simulink library "Miscellaneous"  (Simulink 8.7)
settings: Solver=ode45  StartTime=0.0  StopTime=10.0  RelTol=1e-3
undefined symbols (not defined in the file): c
libraries: Memory_Blocks_Lib x100, Bit_Multiplexers_Lib x35, simulink_extras x13, commutil2 x10, Decoders_Lib x7
settings Model: Creator=N  LastModifiedBy=Jozko Mrkvicka

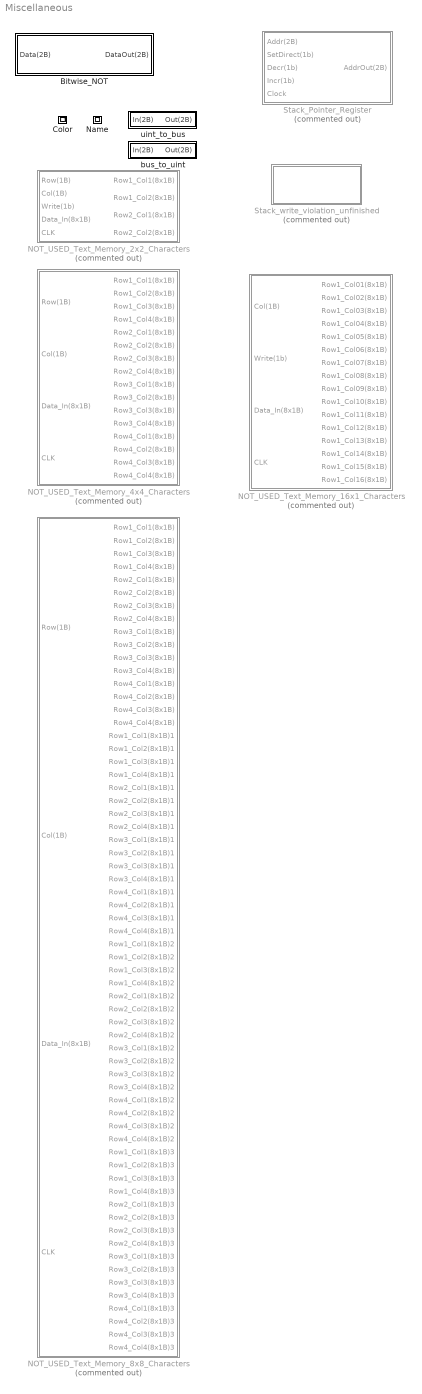
== system Miscellaneous ==
  Bitwise_NOT : Subsystem
  Color : Subsystem
  NOT_USED_Text_Memory_16x1_Characters : Subsystem  Commented=on
  NOT_USED_Text_Memory_2x2_Characters : Subsystem  Commented=on
  NOT_USED_Text_Memory_4x4_Characters : Subsystem  Commented=on
  NOT_USED_Text_Memory_8x8_Characters : Subsystem  Commented=on
  Name : Subsystem
  Stack_Pointer_Register : Subsystem  Commented=on
  Stack_write_violation_unfinished : Subsystem  Commented=on
  bus_to_uint : Subsystem
  uint_to_bus : Subsystem

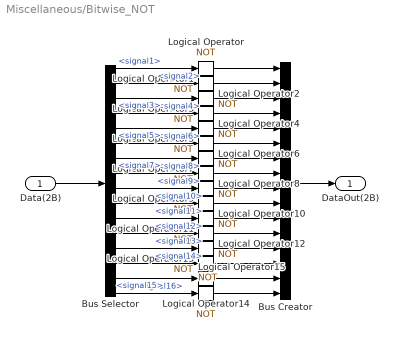
== system Miscellaneous/Bitwise_NOT ==
  Data(2B) : Inport
  Bus Creator : BusCreator  Inputs=16
  Bus Selector : BusSelector  OutputSignals=signal1,signal2,signal3,signal4,signal5,signal6,signal7,signal8,signal9,signal10,signal11,signal12,signal13,signal14,signal15,signal16
  Logical Operator{,1..15} (16 alike) : Logic  Operator=NOT  IconShape=distinctive  AllPortsSameDT=off  OutDataTypeStr=boolean
  DataOut(2B) : Outport
  wires:
  Bus Creator/1 -> DataOut(2B)/1
  Data(2B)/1 -> Bus Selector/1
  Logical Operator/1 -> Bus Creator/1
  Logical Operator1/1 -> Bus Creator/2
  Logical Operator2/1 -> Bus Creator/3
  Logical Operator7/1 -> Bus Creator/8
  Logical Operator6/1 -> Bus Creator/7
  Logical Operator5/1 -> Bus Creator/6
  Logical Operator3/1 -> Bus Creator/4
  Logical Operator4/1 -> Bus Creator/5
  Bus Selector/8 -> Logical Operator7/1  "<signal8>"
  Bus Selector/7 -> Logical Operator6/1  "<signal7>"
  Bus Selector/6 -> Logical Operator5/1  "<signal6>"
  Bus Selector/5 -> Logical Operator4/1  "<signal5>"
  Bus Selector/4 -> Logical Operator3/1  "<signal4>"
  Bus Selector/3 -> Logical Operator2/1  "<signal3>"
  Bus Selector/2 -> Logical Operator1/1  "<signal2>"
  Bus Selector/1 -> Logical Operator/1  "<signal1>"
  Bus Selector/16 -> Logical Operator15/1  "<signal16>"
  Bus Selector/15 -> Logical Operator14/1  "<signal15>"
  Bus Selector/14 -> Logical Operator13/1  "<signal14>"
  Bus Selector/13 -> Logical Operator12/1  "<signal13>"
  Bus Selector/12 -> Logical Operator11/1  "<signal12>"
  Bus Selector/11 -> Logical Operator10/1  "<signal11>"
  Bus Selector/10 -> Logical Operator9/1  "<signal10>"
  Bus Selector/9 -> Logical Operator8/1  "<signal9>"
  Logical Operator8/1 -> Bus Creator/9
  Logical Operator9/1 -> Bus Creator/10
  Logical Operator10/1 -> Bus Creator/11
  Logical Operator11/1 -> Bus Creator/12
  Logical Operator12/1 -> Bus Creator/13
  Logical Operator13/1 -> Bus Creator/14
  Logical Operator14/1 -> Bus Creator/15
  Logical Operator15/1 -> Bus Creator/16

== system Miscellaneous/Color ==
  note: This block is just a workaround for changing color of a line which is connected to it (Simulink does not allow to assign colors to particular lines).
  " " : Inport
  "  " : Outport
  wires:
  " "/1 -> "  "/1

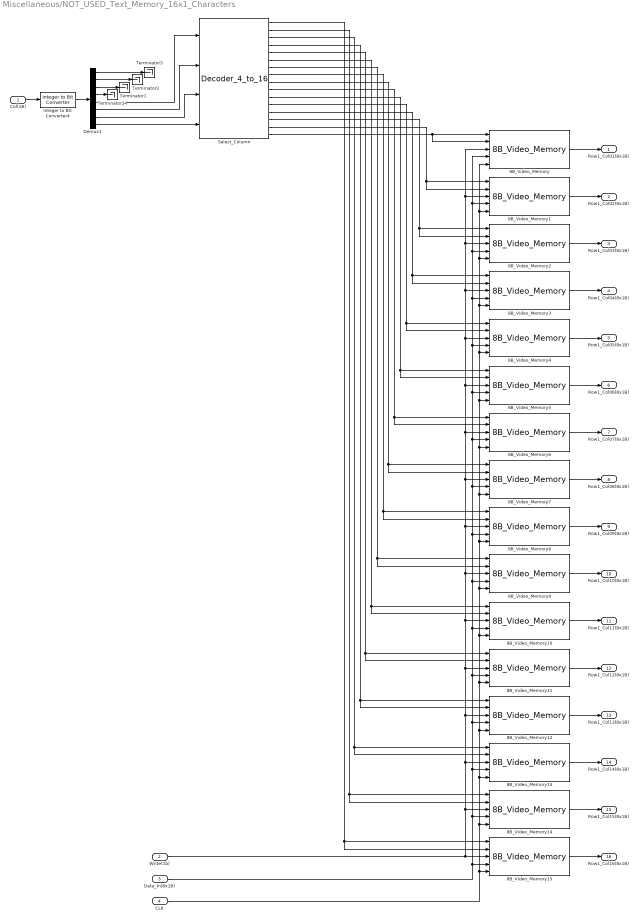
== system Miscellaneous/NOT_USED_Text_Memory_16x1_Characters ==
  Col(1B) : Inport
  Write(1b) : Inport  Port=2
  Data_In(8x1B) : Inport  Port=3
  CLK : Inport  Port=4
  8B_Video_Memory{,1..15} (16 alike) : Memory_Blocks_Lib/Memory_Blocks_Lib/8B_Video_Memory
  Demux1 : Demux  Outputs=8
  Integer to Bit Converter4 : commutil2/Integer to Bit Converter  nbits=8  signedInputValues=Unsigned  bitOrder=MSB first  outDtype=uint8
  Select_Column : Decoders_Lib/Decoders_Lib/Decoder_4_to_16
  Terminator{1..3,24} (4 alike) : Terminator
  Row1_Col01(8x1B) : Outport
  Row1_Col02(8x1B) : Outport  Port=2
  Row1_Col03(8x1B) : Outport  Port=3
  Row1_Col04(8x1B) : Outport  Port=4
  Row1_Col05(8x1B) : Outport  Port=5
  Row1_Col06(8x1B) : Outport  Port=6
  Row1_Col07(8x1B) : Outport  Port=7
  Row1_Col08(8x1B) : Outport  Port=8
  Row1_Col09(8x1B) : Outport  Port=9
  Row1_Col10(8x1B) : Outport  Port=10
  Row1_Col11(8x1B) : Outport  Port=11
  Row1_Col12(8x1B) : Outport  Port=12
  Row1_Col13(8x1B) : Outport  Port=13
  Row1_Col14(8x1B) : Outport  Port=14
  Row1_Col15(8x1B) : Outport  Port=15
  Row1_Col16(8x1B) : Outport  Port=16
  wires:
  Col(1B)/1 -> Integer to Bit Converter4/1
  Integer to Bit Converter4/1 -> Demux1/1
  Data_In(8x1B)/1 -> 8B_Video_Memory6/4, 8B_Video_Memory5/4, 8B_Video_Memory4/4, 8B_Video_Memory3/4, 8B_Video_Memory2/4, 8B_Video_Memory/4, 8B_Video_Memory1/4, 8B_Video_Memory7/4, 8B_Video_Memory8/4, 8B_Video_Memory9/4, 8B_Video_Memory10/4, 8B_Video_Memory11/4, 8B_Video_Memory12/4, 8B_Video_Memory13/4, 8B_Video_Memory14/4, 8B_Video_Memory15/4
  8B_Video_Memory/1 -> Row1_Col01(8x1B)/1
  8B_Video_Memory1/1 -> Row1_Col02(8x1B)/1
  8B_Video_Memory2/1 -> Row1_Col03(8x1B)/1
  8B_Video_Memory3/1 -> Row1_Col04(8x1B)/1
  CLK/1 -> 8B_Video_Memory6/5, 8B_Video_Memory5/5, 8B_Video_Memory4/5, 8B_Video_Memory3/5, 8B_Video_Memory2/5, 8B_Video_Memory/5, 8B_Video_Memory1/5, 8B_Video_Memory7/5, 8B_Video_Memory8/5, 8B_Video_Memory9/5, 8B_Video_Memory10/5, 8B_Video_Memory11/5, 8B_Video_Memory12/5, 8B_Video_Memory13/5, 8B_Video_Memory14/5, 8B_Video_Memory15/5
  8B_Video_Memory4/1 -> Row1_Col05(8x1B)/1
  8B_Video_Memory5/1 -> Row1_Col06(8x1B)/1
  8B_Video_Memory6/1 -> Row1_Col07(8x1B)/1
  8B_Video_Memory7/1 -> Row1_Col08(8x1B)/1
  8B_Video_Memory8/1 -> Row1_Col09(8x1B)/1
  8B_Video_Memory9/1 -> Row1_Col10(8x1B)/1
  8B_Video_Memory10/1 -> Row1_Col11(8x1B)/1
  8B_Video_Memory11/1 -> Row1_Col12(8x1B)/1
  8B_Video_Memory12/1 -> Row1_Col13(8x1B)/1
  8B_Video_Memory13/1 -> Row1_Col14(8x1B)/1
  8B_Video_Memory14/1 -> Row1_Col15(8x1B)/1
  8B_Video_Memory15/1 -> Row1_Col16(8x1B)/1
  Demux1/5 -> Select_Column/1
  Demux1/6 -> Select_Column/2
  Demux1/8 -> Select_Column/4
  Demux1/7 -> Select_Column/3
  Select_Column/16 -> 8B_Video_Memory/2, 8B_Video_Memory/1
  Select_Column/15 -> 8B_Video_Memory1/2, 8B_Video_Memory1/1
  Write(1b)/1 -> 8B_Video_Memory/3, 8B_Video_Memory1/3, 8B_Video_Memory2/3, 8B_Video_Memory3/3, 8B_Video_Memory4/3, 8B_Video_Memory5/3, 8B_Video_Memory6/3, 8B_Video_Memory7/3, 8B_Video_Memory8/3, 8B_Video_Memory9/3, 8B_Video_Memory10/3, 8B_Video_Memory11/3, 8B_Video_Memory12/3, 8B_Video_Memory13/3, 8B_Video_Memory14/3, 8B_Video_Memory15/3
  Select_Column/14 -> 8B_Video_Memory2/2, 8B_Video_Memory2/1
  Select_Column/13 -> 8B_Video_Memory3/1, 8B_Video_Memory3/2
  Select_Column/12 -> 8B_Video_Memory4/1, 8B_Video_Memory4/2
  Select_Column/11 -> 8B_Video_Memory5/1, 8B_Video_Memory5/2
  Select_Column/10 -> 8B_Video_Memory6/1, 8B_Video_Memory6/2
  Select_Column/9 -> 8B_Video_Memory7/1, 8B_Video_Memory7/2
  Select_Column/8 -> 8B_Video_Memory8/1, 8B_Video_Memory8/2
  Select_Column/7 -> 8B_Video_Memory9/1, 8B_Video_Memory9/2
  Select_Column/6 -> 8B_Video_Memory10/1, 8B_Video_Memory10/2
  Select_Column/5 -> 8B_Video_Memory11/1, 8B_Video_Memory11/2
  Select_Column/4 -> 8B_Video_Memory12/1, 8B_Video_Memory12/2
  Select_Column/3 -> 8B_Video_Memory13/1, 8B_Video_Memory13/2
  Select_Column/2 -> 8B_Video_Memory14/1, 8B_Video_Memory14/2
  Select_Column/1 -> 8B_Video_Memory15/1, 8B_Video_Memory15/2
  Demux1/4 -> Terminator24/1
  Demux1/3 -> Terminator1/1
  Demux1/2 -> Terminator2/1
  Demux1/1 -> Terminator3/1

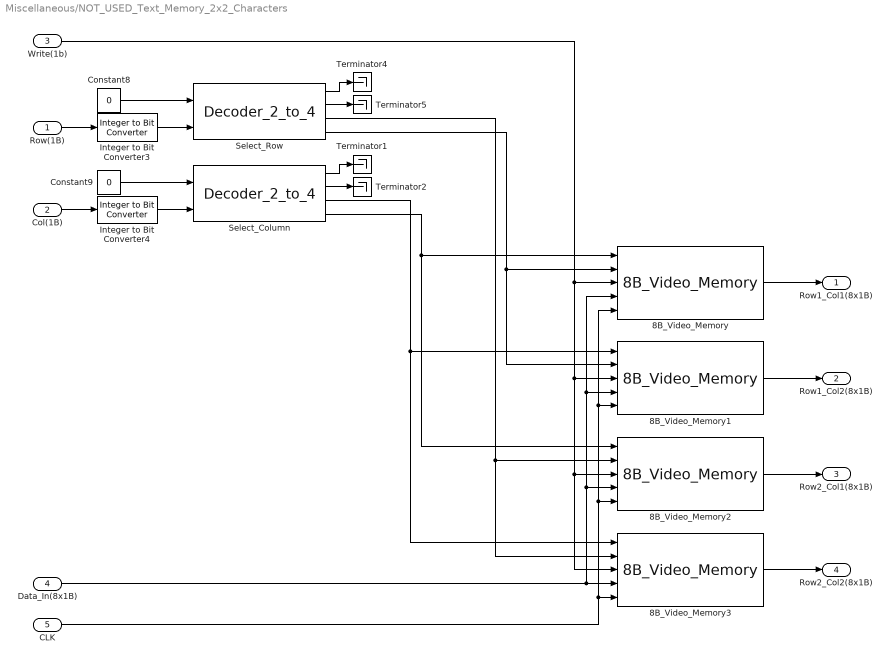
== system Miscellaneous/NOT_USED_Text_Memory_2x2_Characters ==
  Row(1B) : Inport
  Col(1B) : Inport  Port=2
  Write(1b) : Inport  Port=3
  Data_In(8x1B) : Inport  Port=4
  CLK : Inport  Port=5
  8B_Video_Memory{,1..3} (4 alike) : Memory_Blocks_Lib/Memory_Blocks_Lib/8B_Video_Memory
  Constant8 : Constant  Value=0  OutDataTypeStr=uint8
  Constant9 : Constant  Value=0  OutDataTypeStr=uint8
  Integer to Bit Converter3 : commutil2/Integer to Bit Converter  nbits=1  signedInputValues=Unsigned  bitOrder=MSB first  outDtype=uint8
  Integer to Bit Converter4 : commutil2/Integer to Bit Converter  nbits=1  signedInputValues=Unsigned  bitOrder=MSB first  outDtype=uint8
  Select_Column : Decoders_Lib/Decoders_Lib/Decoder_2_to_4
  Select_Row : Decoders_Lib/Decoders_Lib/Decoder_2_to_4
  Terminator{1..2,4..5} (4 alike) : Terminator
  Row1_Col1(8x1B) : Outport
  Row1_Col2(8x1B) : Outport  Port=2
  Row2_Col1(8x1B) : Outport  Port=3
  Row2_Col2(8x1B) : Outport  Port=4
  wires:
  Row(1B)/1 -> Integer to Bit Converter3/1
  Integer to Bit Converter3/1 -> Select_Row/2
  Constant8/1 -> Select_Row/1
  Constant9/1 -> Select_Column/1
  Col(1B)/1 -> Integer to Bit Converter4/1
  Integer to Bit Converter4/1 -> Select_Column/2
  Data_In(8x1B)/1 -> 8B_Video_Memory/4, 8B_Video_Memory1/4, 8B_Video_Memory2/4, 8B_Video_Memory3/4
  8B_Video_Memory/1 -> Row1_Col1(8x1B)/1
  8B_Video_Memory1/1 -> Row1_Col2(8x1B)/1
  8B_Video_Memory2/1 -> Row2_Col1(8x1B)/1
  8B_Video_Memory3/1 -> Row2_Col2(8x1B)/1
  CLK/1 -> 8B_Video_Memory/5, 8B_Video_Memory1/5, 8B_Video_Memory2/5, 8B_Video_Memory3/5
  Select_Row/1 -> Terminator4/1
  Select_Row/2 -> Terminator5/1
  Select_Column/1 -> Terminator1/1
  Select_Column/2 -> Terminator2/1
  Select_Row/4 -> 8B_Video_Memory1/2, 8B_Video_Memory/2
  Select_Row/3 -> 8B_Video_Memory3/2, 8B_Video_Memory2/2
  Select_Column/4 -> 8B_Video_Memory2/1, 8B_Video_Memory/1
  Select_Column/3 -> 8B_Video_Memory3/1, 8B_Video_Memory1/1
  Write(1b)/1 -> 8B_Video_Memory/3, 8B_Video_Memory1/3, 8B_Video_Memory2/3, 8B_Video_Memory3/3

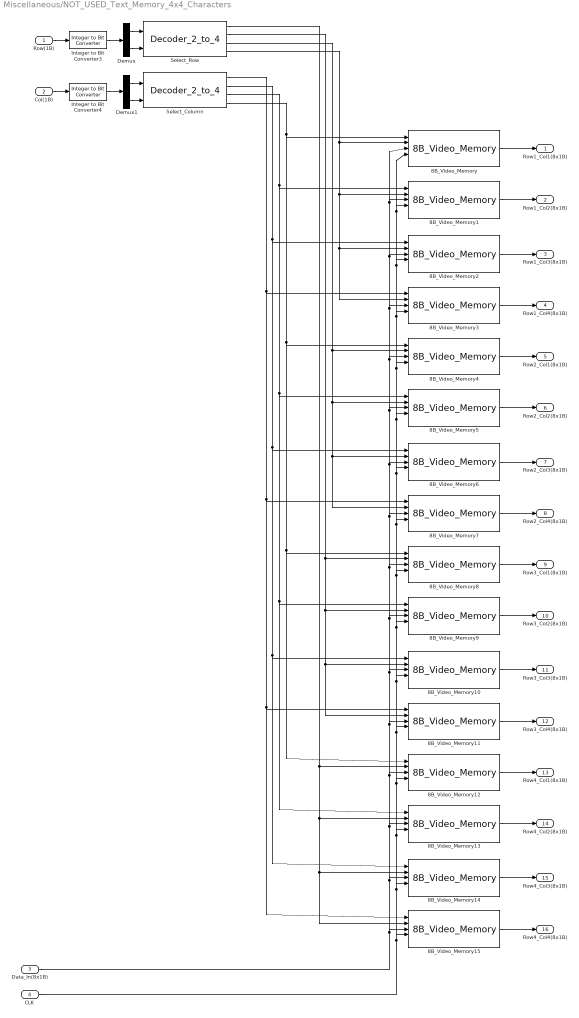
== system Miscellaneous/NOT_USED_Text_Memory_4x4_Characters ==
  Row(1B) : Inport
  Col(1B) : Inport  Port=2
  Data_In(8x1B) : Inport  Port=3
  CLK : Inport  Port=4
  8B_Video_Memory{,1..15} (16 alike) : Memory_Blocks_Lib/Memory_Blocks_Lib/8B_Video_Memory
  Demux : Demux  Outputs=2
  Demux1 : Demux  Outputs=2
  Integer to Bit Converter3 : commutil2/Integer to Bit Converter  nbits=2  signedInputValues=Unsigned  bitOrder=MSB first  outDtype=uint8
  Integer to Bit Converter4 : commutil2/Integer to Bit Converter  nbits=2  signedInputValues=Unsigned  bitOrder=MSB first  outDtype=uint8
  Select_Column : Decoders_Lib/Decoders_Lib/Decoder_2_to_4
  Select_Row : Decoders_Lib/Decoders_Lib/Decoder_2_to_4
  Row1_Col1(8x1B) : Outport
  Row1_Col2(8x1B) : Outport  Port=2
  Row1_Col3(8x1B) : Outport  Port=3
  Row1_Col4(8x1B) : Outport  Port=4
  Row2_Col1(8x1B) : Outport  Port=5
  Row2_Col2(8x1B) : Outport  Port=6
  Row2_Col3(8x1B) : Outport  Port=7
  Row2_Col4(8x1B) : Outport  Port=8
  Row3_Col1(8x1B) : Outport  Port=9
  Row3_Col2(8x1B) : Outport  Port=10
  Row3_Col3(8x1B) : Outport  Port=11
  Row3_Col4(8x1B) : Outport  Port=12
  Row4_Col1(8x1B) : Outport  Port=13
  Row4_Col2(8x1B) : Outport  Port=14
  Row4_Col3(8x1B) : Outport  Port=15
  Row4_Col4(8x1B) : Outport  Port=16
  wires:
  Row(1B)/1 -> Integer to Bit Converter3/1
  Integer to Bit Converter3/1 -> Demux/1
  Col(1B)/1 -> Integer to Bit Converter4/1
  Integer to Bit Converter4/1 -> Demux1/1
  Data_In(8x1B)/1 -> 8B_Video_Memory15/3, 8B_Video_Memory14/3, 8B_Video_Memory13/3, 8B_Video_Memory12/3, 8B_Video_Memory11/3, 8B_Video_Memory10/3, 8B_Video_Memory9/3, 8B_Video_Memory8/3, 8B_Video_Memory6/3, 8B_Video_Memory5/3, 8B_Video_Memory4/3, 8B_Video_Memory2/3, 8B_Video_Memory1/3, 8B_Video_Memory/3, 8B_Video_Memory3/3, 8B_Video_Memory7/3
  8B_Video_Memory/1 -> Row1_Col1(8x1B)/1
  8B_Video_Memory1/1 -> Row1_Col2(8x1B)/1
  8B_Video_Memory2/1 -> Row1_Col3(8x1B)/1
  8B_Video_Memory3/1 -> Row1_Col4(8x1B)/1
  CLK/1 -> 8B_Video_Memory15/4, 8B_Video_Memory14/4, 8B_Video_Memory13/4, 8B_Video_Memory12/4, 8B_Video_Memory11/4, 8B_Video_Memory10/4, 8B_Video_Memory9/4, 8B_Video_Memory8/4, 8B_Video_Memory7/4, 8B_Video_Memory6/4, 8B_Video_Memory5/4, 8B_Video_Memory4/4, 8B_Video_Memory3/4, 8B_Video_Memory2/4, 8B_Video_Memory1/4, 8B_Video_Memory/4
  Select_Row/1 -> 8B_Video_Memory12/2, 8B_Video_Memory13/2, 8B_Video_Memory14/2, 8B_Video_Memory15/2
  Select_Row/2 -> 8B_Video_Memory8/2, 8B_Video_Memory9/2, 8B_Video_Memory10/2, 8B_Video_Memory11/2
  Select_Column/1 -> 8B_Video_Memory15/1, 8B_Video_Memory11/1, 8B_Video_Memory7/1, 8B_Video_Memory3/1
  Select_Column/2 -> 8B_Video_Memory14/1, 8B_Video_Memory10/1, 8B_Video_Memory6/1, 8B_Video_Memory2/1
  Select_Row/4 -> 8B_Video_Memory/2, 8B_Video_Memory1/2, 8B_Video_Memory2/2, 8B_Video_Memory3/2
  Select_Row/3 -> 8B_Video_Memory4/2, 8B_Video_Memory5/2, 8B_Video_Memory6/2, 8B_Video_Memory7/2
  Select_Column/4 -> 8B_Video_Memory12/1, 8B_Video_Memory8/1, 8B_Video_Memory4/1, 8B_Video_Memory/1
  Select_Column/3 -> 8B_Video_Memory13/1, 8B_Video_Memory9/1, 8B_Video_Memory5/1, 8B_Video_Memory1/1
  8B_Video_Memory4/1 -> Row2_Col1(8x1B)/1
  8B_Video_Memory5/1 -> Row2_Col2(8x1B)/1
  8B_Video_Memory6/1 -> Row2_Col3(8x1B)/1
  8B_Video_Memory7/1 -> Row2_Col4(8x1B)/1
  8B_Video_Memory8/1 -> Row3_Col1(8x1B)/1
  8B_Video_Memory9/1 -> Row3_Col2(8x1B)/1
  8B_Video_Memory10/1 -> Row3_Col3(8x1B)/1
  8B_Video_Memory11/1 -> Row3_Col4(8x1B)/1
  8B_Video_Memory12/1 -> Row4_Col1(8x1B)/1
  8B_Video_Memory13/1 -> Row4_Col2(8x1B)/1
  8B_Video_Memory14/1 -> Row4_Col3(8x1B)/1
  8B_Video_Memory15/1 -> Row4_Col4(8x1B)/1
  Demux/1 -> Select_Row/1
  Demux/2 -> Select_Row/2
  Demux1/1 -> Select_Column/1
  Demux1/2 -> Select_Column/2

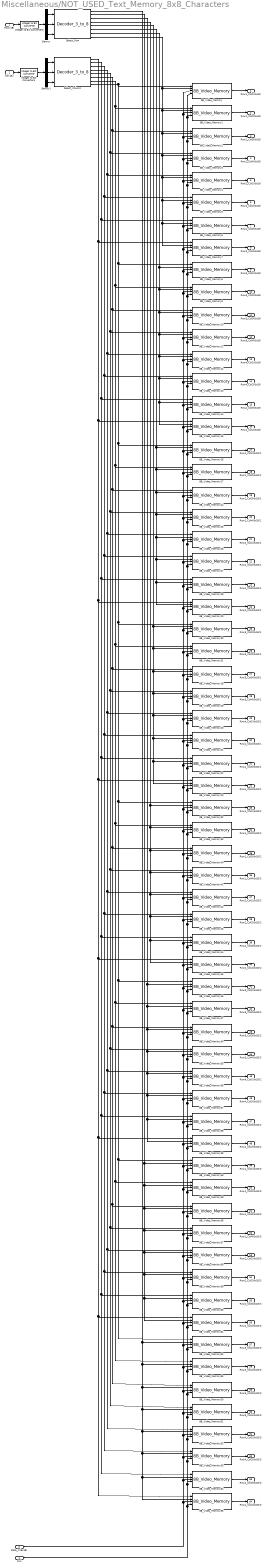
== system Miscellaneous/NOT_USED_Text_Memory_8x8_Characters ==
  Row(1B) : Inport
  Col(1B) : Inport  Port=2
  Data_In(8x1B) : Inport  Port=3
  CLK : Inport  Port=4
  8B_Video_Memory{,1..63} (64 alike) : Memory_Blocks_Lib/Memory_Blocks_Lib/8B_Video_Memory
  Demux : Demux  Outputs=3
  Demux1 : Demux  Outputs=3
  Integer to Bit Converter3 : commutil2/Integer to Bit Converter  nbits=3  signedInputValues=Unsigned  bitOrder=MSB first  outDtype=uint8
  Integer to Bit Converter4 : commutil2/Integer to Bit Converter  nbits=3  signedInputValues=Unsigned  bitOrder=MSB first  outDtype=uint8
  Select_Column : Decoders_Lib/Decoders_Lib/Decoder_3_to_8
  Select_Row : Decoders_Lib/Decoders_Lib/Decoder_3_to_8
  Row1_Col1(8x1B) : Outport
  Row1_Col2(8x1B) : Outport  Port=2
  Row1_Col3(8x1B) : Outport  Port=3
  Row1_Col4(8x1B) : Outport  Port=4
  Row2_Col1(8x1B) : Outport  Port=5
  Row2_Col2(8x1B) : Outport  Port=6
  Row2_Col3(8x1B) : Outport  Port=7
  Row2_Col4(8x1B) : Outport  Port=8
  Row3_Col1(8x1B) : Outport  Port=9
  Row3_Col2(8x1B) : Outport  Port=10
  Row3_Col3(8x1B) : Outport  Port=11
  Row3_Col4(8x1B) : Outport  Port=12
  Row4_Col1(8x1B) : Outport  Port=13
  Row4_Col2(8x1B) : Outport  Port=14
  Row4_Col3(8x1B) : Outport  Port=15
  Row4_Col4(8x1B) : Outport  Port=16
  Row1_Col1(8x1B)1 : Outport  Port=17
  Row1_Col2(8x1B)1 : Outport  Port=18
  Row1_Col3(8x1B)1 : Outport  Port=19
  Row1_Col4(8x1B)1 : Outport  Port=20
  Row2_Col1(8x1B)1 : Outport  Port=21
  Row2_Col2(8x1B)1 : Outport  Port=22
  Row2_Col3(8x1B)1 : Outport  Port=23
  Row2_Col4(8x1B)1 : Outport  Port=24
  Row3_Col1(8x1B)1 : Outport  Port=25
  Row3_Col2(8x1B)1 : Outport  Port=26
  Row3_Col3(8x1B)1 : Outport  Port=27
  Row3_Col4(8x1B)1 : Outport  Port=28
  Row4_Col1(8x1B)1 : Outport  Port=29
  Row4_Col2(8x1B)1 : Outport  Port=30
  Row4_Col3(8x1B)1 : Outport  Port=31
  Row4_Col4(8x1B)1 : Outport  Port=32
  Row1_Col1(8x1B)2 : Outport  Port=33
  Row1_Col2(8x1B)2 : Outport  Port=34
  Row1_Col3(8x1B)2 : Outport  Port=35
  Row1_Col4(8x1B)2 : Outport  Port=36
  Row2_Col1(8x1B)2 : Outport  Port=37
  Row2_Col2(8x1B)2 : Outport  Port=38
  Row2_Col3(8x1B)2 : Outport  Port=39
  Row2_Col4(8x1B)2 : Outport  Port=40
  Row3_Col1(8x1B)2 : Outport  Port=41
  Row3_Col2(8x1B)2 : Outport  Port=42
  Row3_Col3(8x1B)2 : Outport  Port=43
  Row3_Col4(8x1B)2 : Outport  Port=44
  Row4_Col1(8x1B)2 : Outport  Port=45
  Row4_Col2(8x1B)2 : Outport  Port=46
  Row4_Col3(8x1B)2 : Outport  Port=47
  Row4_Col4(8x1B)2 : Outport  Port=48
  Row1_Col1(8x1B)3 : Outport  Port=49
  Row1_Col2(8x1B)3 : Outport  Port=50
  Row1_Col3(8x1B)3 : Outport  Port=51
  Row1_Col4(8x1B)3 : Outport  Port=52
  Row2_Col1(8x1B)3 : Outport  Port=53
  Row2_Col2(8x1B)3 : Outport  Port=54
  Row2_Col3(8x1B)3 : Outport  Port=55
  Row2_Col4(8x1B)3 : Outport  Port=56
  Row3_Col1(8x1B)3 : Outport  Port=57
  Row3_Col2(8x1B)3 : Outport  Port=58
  Row3_Col3(8x1B)3 : Outport  Port=59
  Row3_Col4(8x1B)3 : Outport  Port=60
  Row4_Col1(8x1B)3 : Outport  Port=61
  Row4_Col2(8x1B)3 : Outport  Port=62
  Row4_Col3(8x1B)3 : Outport  Port=63
  Row4_Col4(8x1B)3 : Outport  Port=64
  wires:
  Row(1B)/1 -> Integer to Bit Converter3/1
  Integer to Bit Converter3/1 -> Demux/1
  Col(1B)/1 -> Integer to Bit Converter4/1
  Integer to Bit Converter4/1 -> Demux1/1
  8B_Video_Memory/1 -> Row1_Col1(8x1B)/1
  8B_Video_Memory1/1 -> Row1_Col2(8x1B)/1
  8B_Video_Memory2/1 -> Row1_Col3(8x1B)/1
  8B_Video_Memory3/1 -> Row1_Col4(8x1B)/1
  Select_Row/5 -> 8B_Video_Memory30/2, 8B_Video_Memory31/2, 8B_Video_Memory18/2, 8B_Video_Memory19/2, 8B_Video_Memory20/2, 8B_Video_Memory21/2, 8B_Video_Memory22/2, 8B_Video_Memory23/2
  Select_Row/6 -> 8B_Video_Memory16/2, 8B_Video_Memory17/2, 8B_Video_Memory24/2, 8B_Video_Memory25/2, 8B_Video_Memory26/2, 8B_Video_Memory27/2, 8B_Video_Memory28/2, 8B_Video_Memory29/2
  Select_Column/5 -> 8B_Video_Memory3/1, 8B_Video_Memory51/1, 8B_Video_Memory57/1, 8B_Video_Memory35/1, 8B_Video_Memory41/1, 8B_Video_Memory19/1, 8B_Video_Memory25/1, 8B_Video_Memory11/1
  Select_Column/6 -> 8B_Video_Memory2/1, 8B_Video_Memory50/1, 8B_Video_Memory56/1, 8B_Video_Memory34/1, 8B_Video_Memory40/1, 8B_Video_Memory18/1, 8B_Video_Memory24/1, 8B_Video_Memory10/1
  Select_Row/8 -> 8B_Video_Memory/2, 8B_Video_Memory1/2, 8B_Video_Memory2/2, 8B_Video_Memory3/2, 8B_Video_Memory4/2, 8B_Video_Memory5/2, 8B_Video_Memory6/2, 8B_Video_Memory7/2
  Select_Row/7 -> 8B_Video_Memory8/2, 8B_Video_Memory9/2, 8B_Video_Memory10/2, 8B_Video_Memory11/2, 8B_Video_Memory12/2, 8B_Video_Memory13/2, 8B_Video_Memory14/2, 8B_Video_Memory15/2
  Select_Column/8 -> 8B_Video_Memory/1, 8B_Video_Memory62/1, 8B_Video_Memory48/1, 8B_Video_Memory46/1, 8B_Video_Memory32/1, 8B_Video_Memory30/1, 8B_Video_Memory16/1, 8B_Video_Memory8/1
  Select_Column/7 -> 8B_Video_Memory1/1, 8B_Video_Memory63/1, 8B_Video_Memory49/1, 8B_Video_Memory47/1, 8B_Video_Memory33/1, 8B_Video_Memory31/1, 8B_Video_Memory17/1, 8B_Video_Memory9/1
  8B_Video_Memory4/1 -> Row2_Col1(8x1B)/1
  8B_Video_Memory5/1 -> Row2_Col2(8x1B)/1
  8B_Video_Memory6/1 -> Row2_Col3(8x1B)/1
  8B_Video_Memory7/1 -> Row2_Col4(8x1B)/1
  8B_Video_Memory8/1 -> Row3_Col1(8x1B)/1
  8B_Video_Memory9/1 -> Row3_Col2(8x1B)/1
  8B_Video_Memory10/1 -> Row3_Col3(8x1B)/1
  8B_Video_Memory11/1 -> Row3_Col4(8x1B)/1
  8B_Video_Memory12/1 -> Row4_Col1(8x1B)/1
  8B_Video_Memory13/1 -> Row4_Col2(8x1B)/1
  8B_Video_Memory14/1 -> Row4_Col3(8x1B)/1
  8B_Video_Memory15/1 -> Row4_Col4(8x1B)/1
  Demux/1 -> Select_Row/1
  Demux/2 -> Select_Row/2
  Demux1/1 -> Select_Column/1
  Demux1/2 -> Select_Column/2
  8B_Video_Memory16/1 -> Row1_Col1(8x1B)1/1
  8B_Video_Memory17/1 -> Row1_Col2(8x1B)1/1
  8B_Video_Memory24/1 -> Row1_Col3(8x1B)1/1
  8B_Video_Memory25/1 -> Row1_Col4(8x1B)1/1
  8B_Video_Memory26/1 -> Row2_Col1(8x1B)1/1
  8B_Video_Memory27/1 -> Row2_Col2(8x1B)1/1
  8B_Video_Memory28/1 -> Row2_Col3(8x1B)1/1
  8B_Video_Memory29/1 -> Row2_Col4(8x1B)1/1
  8B_Video_Memory30/1 -> Row3_Col1(8x1B)1/1
  8B_Video_Memory31/1 -> Row3_Col2(8x1B)1/1
  8B_Video_Memory18/1 -> Row3_Col3(8x1B)1/1
  8B_Video_Memory19/1 -> Row3_Col4(8x1B)1/1
  8B_Video_Memory20/1 -> Row4_Col1(8x1B)1/1
  8B_Video_Memory21/1 -> Row4_Col2(8x1B)1/1
  8B_Video_Memory22/1 -> Row4_Col3(8x1B)1/1
  8B_Video_Memory23/1 -> Row4_Col4(8x1B)1/1
  8B_Video_Memory32/1 -> Row1_Col1(8x1B)2/1
  8B_Video_Memory33/1 -> Row1_Col2(8x1B)2/1
  8B_Video_Memory40/1 -> Row1_Col3(8x1B)2/1
  8B_Video_Memory41/1 -> Row1_Col4(8x1B)2/1
  8B_Video_Memory42/1 -> Row2_Col1(8x1B)2/1
  8B_Video_Memory43/1 -> Row2_Col2(8x1B)2/1
  8B_Video_Memory44/1 -> Row2_Col3(8x1B)2/1
  8B_Video_Memory45/1 -> Row2_Col4(8x1B)2/1
  8B_Video_Memory46/1 -> Row3_Col1(8x1B)2/1
  8B_Video_Memory47/1 -> Row3_Col2(8x1B)2/1
  8B_Video_Memory34/1 -> Row3_Col3(8x1B)2/1
  8B_Video_Memory35/1 -> Row3_Col4(8x1B)2/1
  8B_Video_Memory36/1 -> Row4_Col1(8x1B)2/1
  8B_Video_Memory37/1 -> Row4_Col2(8x1B)2/1
  8B_Video_Memory38/1 -> Row4_Col3(8x1B)2/1
  8B_Video_Memory39/1 -> Row4_Col4(8x1B)2/1
  8B_Video_Memory48/1 -> Row1_Col1(8x1B)3/1
  8B_Video_Memory49/1 -> Row1_Col2(8x1B)3/1
  8B_Video_Memory56/1 -> Row1_Col3(8x1B)3/1
  8B_Video_Memory57/1 -> Row1_Col4(8x1B)3/1
  8B_Video_Memory58/1 -> Row2_Col1(8x1B)3/1
  8B_Video_Memory59/1 -> Row2_Col2(8x1B)3/1
  8B_Video_Memory60/1 -> Row2_Col3(8x1B)3/1
  8B_Video_Memory61/1 -> Row2_Col4(8x1B)3/1
  8B_Video_Memory62/1 -> Row3_Col1(8x1B)3/1
  8B_Video_Memory63/1 -> Row3_Col2(8x1B)3/1
  8B_Video_Memory50/1 -> Row3_Col3(8x1B)3/1
  8B_Video_Memory51/1 -> Row3_Col4(8x1B)3/1
  8B_Video_Memory52/1 -> Row4_Col1(8x1B)3/1
  8B_Video_Memory53/1 -> Row4_Col2(8x1B)3/1
  8B_Video_Memory54/1 -> Row4_Col3(8x1B)3/1
  8B_Video_Memory55/1 -> Row4_Col4(8x1B)3/1
  Data_In(8x1B)/1 -> 8B_Video_Memory55/3, 8B_Video_Memory54/3, 8B_Video_Memory53/3, 8B_Video_Memory52/3, 8B_Video_Memory51/3, 8B_Video_Memory50/3, 8B_Video_Memory63/3, 8B_Video_Memory62/3, 8B_Video_Memory61/3, 8B_Video_Memory60/3, 8B_Video_Memory59/3, 8B_Video_Memory58/3, 8B_Video_Memory57/3, 8B_Video_Memory56/3, 8B_Video_Memory49/3, 8B_Video_Memory48/3, 8B_Video_Memory39/3, 8B_Video_Memory38/3, 8B_Video_Memory37/3, 8B_Video_Memory36/3, 8B_Video_Memory35/3, 8B_Video_Memory34/3, 8B_Video_Memory47/3, 8B_Video_Memory46/3, 8B_Video_Memory45/3, 8B_Video_Memory44/3, 8B_Video_Memory43/3, 8B_Video_Memory42/3, 8B_Video_Memory41/3, 8B_Video_Memory40/3, 8B_Video_Memory33/3, 8B_Video_Memory32/3, 8B_Video_Memory23/3, 8B_Video_Memory22/3, 8B_Video_Memory21/3, 8B_Video_Memory20/3, 8B_Video_Memory19/3, 8B_Video_Memory18/3, 8B_Video_Memory31/3, 8B_Video_Memory30/3, 8B_Video_Memory29/3, 8B_Video_Memory28/3, 8B_Video_Memory27/3, 8B_Video_Memory26/3, 8B_Video_Memory25/3, 8B_Video_Memory24/3, 8B_Video_Memory17/3, 8B_Video_Memory16/3, 8B_Video_Memory15/3, 8B_Video_Memory14/3, 8B_Video_Memory13/3, 8B_Video_Memory12/3, 8B_Video_Memory11/3, 8B_Video_Memory10/3, 8B_Video_Memory9/3, 8B_Video_Memory8/3, 8B_Video_Memory6/3, 8B_Video_Memory5/3, 8B_Video_Memory4/3, 8B_Video_Memory2/3, 8B_Video_Memory1/3, 8B_Video_Memory/3, 8B_Video_Memory3/3, 8B_Video_Memory7/3
  CLK/1 -> 8B_Video_Memory55/4, 8B_Video_Memory54/4, 8B_Video_Memory53/4, 8B_Video_Memory52/4, 8B_Video_Memory51/4, 8B_Video_Memory50/4, 8B_Video_Memory63/4, 8B_Video_Memory62/4, 8B_Video_Memory61/4, 8B_Video_Memory60/4, 8B_Video_Memory59/4, 8B_Video_Memory58/4, 8B_Video_Memory57/4, 8B_Video_Memory56/4, 8B_Video_Memory49/4, 8B_Video_Memory48/4, 8B_Video_Memory39/4, 8B_Video_Memory38/4, 8B_Video_Memory37/4, 8B_Video_Memory36/4, 8B_Video_Memory35/4, 8B_Video_Memory34/4, 8B_Video_Memory47/4, 8B_Video_Memory46/4, 8B_Video_Memory45/4, 8B_Video_Memory44/4, 8B_Video_Memory43/4, 8B_Video_Memory42/4, 8B_Video_Memory41/4, 8B_Video_Memory40/4, 8B_Video_Memory33/4, 8B_Video_Memory32/4, 8B_Video_Memory23/4, 8B_Video_Memory22/4, 8B_Video_Memory21/4, 8B_Video_Memory20/4, 8B_Video_Memory19/4, 8B_Video_Memory18/4, 8B_Video_Memory31/4, 8B_Video_Memory30/4, 8B_Video_Memory29/4, 8B_Video_Memory28/4, 8B_Video_Memory27/4, 8B_Video_Memory26/4, 8B_Video_Memory25/4, 8B_Video_Memory24/4, 8B_Video_Memory17/4, 8B_Video_Memory16/4, 8B_Video_Memory15/4, 8B_Video_Memory14/4, 8B_Video_Memory13/4, 8B_Video_Memory12/4, 8B_Video_Memory11/4, 8B_Video_Memory10/4, 8B_Video_Memory9/4, 8B_Video_Memory8/4, 8B_Video_Memory7/4, 8B_Video_Memory6/4, 8B_Video_Memory5/4, 8B_Video_Memory4/4, 8B_Video_Memory3/4, 8B_Video_Memory2/4, 8B_Video_Memory1/4, 8B_Video_Memory/4
  Select_Row/4 -> 8B_Video_Memory32/2, 8B_Video_Memory33/2, 8B_Video_Memory40/2, 8B_Video_Memory41/2, 8B_Video_Memory42/2, 8B_Video_Memory43/2, 8B_Video_Memory44/2, 8B_Video_Memory45/2
  Select_Row/3 -> 8B_Video_Memory46/2, 8B_Video_Memory47/2, 8B_Video_Memory34/2, 8B_Video_Memory35/2, 8B_Video_Memory36/2, 8B_Video_Memory37/2, 8B_Video_Memory38/2, 8B_Video_Memory39/2
  Select_Row/2 -> 8B_Video_Memory48/2, 8B_Video_Memory49/2, 8B_Video_Memory56/2, 8B_Video_Memory57/2, 8B_Video_Memory58/2, 8B_Video_Memory60/2, 8B_Video_Memory61/2, 8B_Video_Memory59/2
  Select_Row/1 -> 8B_Video_Memory62/2, 8B_Video_Memory63/2, 8B_Video_Memory50/2, 8B_Video_Memory51/2, 8B_Video_Memory52/2, 8B_Video_Memory53/2, 8B_Video_Memory54/2, 8B_Video_Memory55/2
  Select_Column/4 -> 8B_Video_Memory52/1, 8B_Video_Memory58/1, 8B_Video_Memory36/1, 8B_Video_Memory42/1, 8B_Video_Memory20/1, 8B_Video_Memory26/1, 8B_Video_Memory12/1, 8B_Video_Memory4/1
  Select_Column/3 -> 8B_Video_Memory53/1, 8B_Video_Memory59/1, 8B_Video_Memory37/1, 8B_Video_Memory43/1, 8B_Video_Memory21/1, 8B_Video_Memory27/1, 8B_Video_Memory13/1, 8B_Video_Memory5/1
  Select_Column/2 -> 8B_Video_Memory54/1, 8B_Video_Memory60/1, 8B_Video_Memory38/1, 8B_Video_Memory44/1, 8B_Video_Memory22/1, 8B_Video_Memory28/1, 8B_Video_Memory14/1, 8B_Video_Memory6/1
  Select_Column/1 -> 8B_Video_Memory55/1, 8B_Video_Memory61/1, 8B_Video_Memory39/1, 8B_Video_Memory45/1, 8B_Video_Memory23/1, 8B_Video_Memory29/1, 8B_Video_Memory15/1, 8B_Video_Memory7/1
  Demux/3 -> Select_Row/3
  Demux1/3 -> Select_Column/3

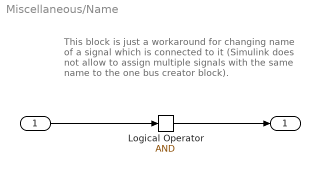
== system Miscellaneous/Name ==
  note: This block is just a workaround for changing name of a signal which is connected to it (Simulink does not allow to assign multiple signals with the same name to the one bus creator block).
  " " : Inport
  Logical Operator : Logic  Inputs=1  IconShape=distinctive  AllPortsSameDT=off  OutDataTypeStr=boolean
  "  " : Outport
  wires:
  " "/1 -> Logical Operator/1
  Logical Operator/1 -> "  "/1

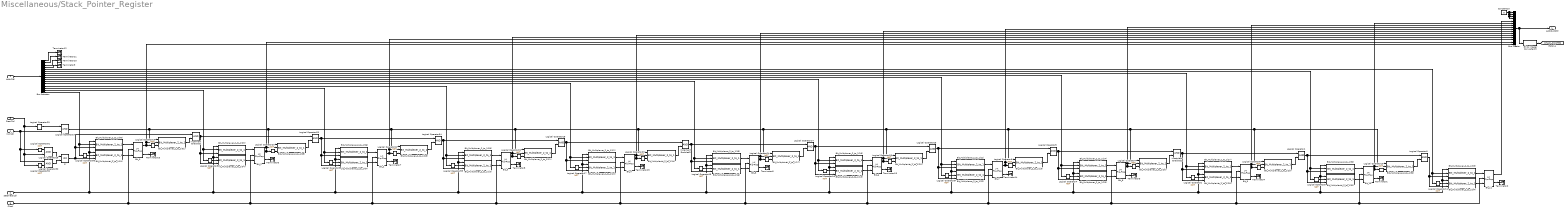
== system Miscellaneous/Stack_Pointer_Register ==
  Addr(2B) : Inport
  SetDirect(1b) : Inport  Port=2
  Decr(1b) : Inport  Port=3
  Incr(1b) : Inport  Port=4
  Clock : Inport  Port=5
  Bit to Integer Converter15 : commutil2/Bit to Integer Converter  nbits=16  bitOrder=MSB first  signedOutputValues=Unsigned  outDtype=uint16  outDtypeSigned=Inherit via internal rule
  Bit_0 : simulink_extras/Flip Flops/J-K Flip-Flop  initial_condition=bitand(c.STACK_START, bin2dec('0000 0000 0001'))
  Bit_1 : simulink_extras/Flip Flops/J-K Flip-Flop  initial_condition=bitand(c.STACK_START, bin2dec('0000 0000 0010'))
  Bit_10 : simulink_extras/Flip Flops/J-K Flip-Flop  initial_condition=bitand(c.STACK_START, bin2dec('0100 0000 0000'))
  Bit_11 : simulink_extras/Flip Flops/J-K Flip-Flop  initial_condition=bitand(c.STACK_START, bin2dec('1000 0000 0000'))
  Bit_2 : simulink_extras/Flip Flops/J-K Flip-Flop  initial_condition=bitand(c.STACK_START, bin2dec('0000 0000 0100'))
  Bit_3 : simulink_extras/Flip Flops/J-K Flip-Flop  initial_condition=bitand(c.STACK_START, bin2dec('0000 0000 1000'))
  Bit_4 : simulink_extras/Flip Flops/J-K Flip-Flop  initial_condition=bitand(c.STACK_START, bin2dec('0000 0001 0000'))
  Bit_5 : simulink_extras/Flip Flops/J-K Flip-Flop  initial_condition=bitand(c.STACK_START, bin2dec('0000 0010 0000'))
  Bit_6 : simulink_extras/Flip Flops/J-K Flip-Flop  initial_condition=bitand(c.STACK_START, bin2dec('0000 0100 0000'))
  Bit_7 : simulink_extras/Flip Flops/J-K Flip-Flop  initial_condition=bitand(c.STACK_START, bin2dec('0000 1000 0000'))
  Bit_8 : simulink_extras/Flip Flops/J-K Flip-Flop  initial_condition=bitand(c.STACK_START, bin2dec('0001 0000 0000'))
  Bit_9 : simulink_extras/Flip Flops/J-K Flip-Flop  initial_condition=bitand(c.STACK_START, bin2dec('0010 0000 0000'))
  Bit_Multiplexer_2_to_1(00) : Bit_Multiplexers_Lib/Bit_Multiplexers_Lib/Bit_Multiplexer_2_to_1
  Bit_Multiplexer_2_to_1(01) : Bit_Multiplexers_Lib/Bit_Multiplexers_Lib/Bit_Multiplexer_2_to_1
  Bit_Multiplexer_2_to_1(02) : Bit_Multiplexers_Lib/Bit_Multiplexers_Lib/Bit_Multiplexer_2_to_1
  Bit_Multiplexer_2_to_1(03) : Bit_Multiplexers_Lib/Bit_Multiplexers_Lib/Bit_Multiplexer_2_to_1
  Bit_Multiplexer_2_to_1(04) : Bit_Multiplexers_Lib/Bit_Multiplexers_Lib/Bit_Multiplexer_2_to_1
  Bit_Multiplexer_2_to_1(05) : Bit_Multiplexers_Lib/Bit_Multiplexers_Lib/Bit_Multiplexer_2_to_1
  Bit_Multiplexer_2_to_1(06) : Bit_Multiplexers_Lib/Bit_Multiplexers_Lib/Bit_Multiplexer_2_to_1
  Bit_Multiplexer_2_to_1(07) : Bit_Multiplexers_Lib/Bit_Multiplexers_Lib/Bit_Multiplexer_2_to_1
  Bit_Multiplexer_2_to_1(08) : Bit_Multiplexers_Lib/Bit_Multiplexers_Lib/Bit_Multiplexer_2_to_1
  Bit_Multiplexer_2_to_1(09) : Bit_Multiplexers_Lib/Bit_Multiplexers_Lib/Bit_Multiplexer_2_to_1
  Bit_Multiplexer_2_to_1(10) : Bit_Multiplexers_Lib/Bit_Multiplexers_Lib/Bit_Multiplexer_2_to_1
  Bit_Multiplexer_2_to_1(11) : Bit_Multiplexers_Lib/Bit_Multiplexers_Lib/Bit_Multiplexer_2_to_1
  Bit_Multiplexer_2_to_1(12) : Bit_Multiplexers_Lib/Bit_Multiplexers_Lib/Bit_Multiplexer_2_to_1
  Bit_Multiplexer_2_to_1(13) : Bit_Multiplexers_Lib/Bit_Multiplexers_Lib/Bit_Multiplexer_2_to_1
  Bit_Multiplexer_2_to_1(14) : Bit_Multiplexers_Lib/Bit_Multiplexers_Lib/Bit_Multiplexer_2_to_1
  Bit_Multiplexer_2_to_1(15) : Bit_Multiplexers_Lib/Bit_Multiplexers_Lib/Bit_Multiplexer_2_to_1
  Bit_Multiplexer_2_to_1(16) : Bit_Multiplexers_Lib/Bit_Multiplexers_Lib/Bit_Multiplexer_2_to_1
  Bit_Multiplexer_2_to_1(17) : Bit_Multiplexers_Lib/Bit_Multiplexers_Lib/Bit_Multiplexer_2_to_1
  Bit_Multiplexer_2_to_1(18) : Bit_Multiplexers_Lib/Bit_Multiplexers_Lib/Bit_Multiplexer_2_to_1
  Bit_Multiplexer_2_to_1(19) : Bit_Multiplexers_Lib/Bit_Multiplexers_Lib/Bit_Multiplexer_2_to_1
  Bit_Multiplexer_2_to_1(20) : Bit_Multiplexers_Lib/Bit_Multiplexers_Lib/Bit_Multiplexer_2_to_1
  Bit_Multiplexer_2_to_1(21) : Bit_Multiplexers_Lib/Bit_Multiplexers_Lib/Bit_Multiplexer_2_to_1
  Bit_Multiplexer_2_to_1(22) : Bit_Multiplexers_Lib/Bit_Multiplexers_Lib/Bit_Multiplexer_2_to_1
  Bit_Multiplexer_2_to_1(23) : Bit_Multiplexers_Lib/Bit_Multiplexers_Lib/Bit_Multiplexer_2_to_1
  Bit_Multiplexer_2_to_1(24) : Bit_Multiplexers_Lib/Bit_Multiplexers_Lib/Bit_Multiplexer_2_to_1
  Bit_Multiplexer_2_to_1(25) : Bit_Multiplexers_Lib/Bit_Multiplexers_Lib/Bit_Multiplexer_2_to_1
  Bit_Multiplexer_2_to_1(26) : Bit_Multiplexers_Lib/Bit_Multiplexers_Lib/Bit_Multiplexer_2_to_1
  Bit_Multiplexer_2_to_1(27) : Bit_Multiplexers_Lib/Bit_Multiplexers_Lib/Bit_Multiplexer_2_to_1
  Bit_Multiplexer_2_to_1(28) : Bit_Multiplexers_Lib/Bit_Multiplexers_Lib/Bit_Multiplexer_2_to_1
  Bit_Multiplexer_2_to_1(29) : Bit_Multiplexers_Lib/Bit_Multiplexers_Lib/Bit_Multiplexer_2_to_1
  Bit_Multiplexer_2_to_1(30) : Bit_Multiplexers_Lib/Bit_Multiplexers_Lib/Bit_Multiplexer_2_to_1
  Bit_Multiplexer_2_to_1(31) : Bit_Multiplexers_Lib/Bit_Multiplexers_Lib/Bit_Multiplexer_2_to_1
  Bit_Multiplexer_2_to_1(32) : Bit_Multiplexers_Lib/Bit_Multiplexers_Lib/Bit_Multiplexer_2_to_1
  Bit_Multiplexer_2_to_1(33) : Bit_Multiplexers_Lib/Bit_Multiplexers_Lib/Bit_Multiplexer_2_to_1
  Bit_Multiplexer_2_to_1(34) : Bit_Multiplexers_Lib/Bit_Multiplexers_Lib/Bit_Multiplexer_2_to_1
  Bus Creator : BusCreator  Inputs=16
  Bus Selector : BusSelector  OutputSignals=signal1,signal2,signal3,signal4,signal5,signal6,signal7,signal8,signal9,signal10,signal11,signal12,signal13,signal14,signal15,signal16
  Constant10 : Constant  Value=0  OutDataTypeStr=boolean
  Increment Enabled1 : Logic  IconShape=distinctive  AllPortsSameDT=off  OutDataTypeStr=boolean
  Increment Enabled2 : Logic  IconShape=distinctive  AllPortsSameDT=off  OutDataTypeStr=boolean
  Increment Enabled3 : Logic  IconShape=distinctive  AllPortsSameDT=off  OutDataTypeStr=boolean
  Logical Operator{1,5,9,14,18,25,27..28,30,33..34} (11 alike) : Logic  IconShape=distinctive  AllPortsSameDT=off  OutDataTypeStr=boolean
  Logical Operator{2..4,6..8,10..11,15..17,19..24,26,29,31..32,35..39} (26 alike) : Logic  Operator=NOT  IconShape=distinctive  AllPortsSameDT=off  OutDataTypeStr=boolean
  Terminator{1..16} (16 alike) : Terminator
  or : Logic  Operator=OR  IconShape=distinctive  AllPortsSameDT=off  OutDataTypeStr=boolean
  AddrOut(2B) : Outport
  tag scope: STACK_POINTER=global
  wires:
  Logical Operator18/1 -> Increment Enabled3/1, Bit_Multiplexer_2_to_1(13)/3, Bit_Multiplexer_2_to_1(12)/3
  Bus Selector/12 -> Bit_Multiplexer_2_to_1(12)/2, Logical Operator17/1  "<signal12>"
  Logical Operator17/1 -> Bit_Multiplexer_2_to_1(13)/2
  Bit_4/1 -> Bus Creator/12, Bit_Multiplexer_2_to_1(14)/2, Logical Operator23/1
  Bus Selector/9 -> Bit_Multiplexer_2_to_1(21)/2, Logical Operator37/1  "<signal9>"
  Logical Operator37/1 -> Bit_Multiplexer_2_to_1(22)/2
  Bit_Multiplexer_2_to_1(21)/1 -> Bit_7/1
  Bit_Multiplexer_2_to_1(22)/1 -> Bit_7/3
  Logical Operator16/1 -> Bit_Multiplexer_2_to_1(19)/2
  Bus Selector/10 -> Bit_Multiplexer_2_to_1(18)/2, Logical Operator16/1  "<signal10>"
  Bit_Multiplexer_2_to_1(19)/1 -> Bit_6/3
  Bit_Multiplexer_2_to_1(18)/1 -> Bit_6/1
  Bus Selector/11 -> Bit_Multiplexer_2_to_1(15)/2, Logical Operator15/1  "<signal11>"
  Logical Operator15/1 -> Bit_Multiplexer_2_to_1(16)/2
  Bit_Multiplexer_2_to_1(16)/1 -> Bit_5/3
  Bit_Multiplexer_2_to_1(15)/1 -> Bit_5/1
  Bit_Multiplexer_2_to_1(12)/1 -> Bit_4/1
  Bit_Multiplexer_2_to_1(13)/1 -> Bit_4/3
  Bit_7/1 -> Bus Creator/9, Bit_Multiplexer_2_to_1(23)/2, Logical Operator6/1
  Bit_6/1 -> Bus Creator/10, Bit_Multiplexer_2_to_1(20)/2, Logical Operator26/1
  Bit_7/2 -> Terminator14/1
  Logical Operator14/1 -> Logical Operator25/1, Bit_Multiplexer_2_to_1(19)/3, Bit_Multiplexer_2_to_1(18)/3
  Bit_5/1 -> Bus Creator/11, Bit_Multiplexer_2_to_1(17)/2, Logical Operator24/1
  Increment Enabled3/1 -> Logical Operator14/1, Bit_Multiplexer_2_to_1(16)/3, Bit_Multiplexer_2_to_1(15)/3
  Bit_6/2 -> Terminator13/1
  Bit_5/2 -> Terminator5/1
  Bit_4/2 -> Terminator15/1
  Logical Operator34/1 -> Logical Operator18/1, Bit_Multiplexer_2_to_1(10)/3, Bit_Multiplexer_2_to_1(09)/3
  Bit_0/1 -> Bus Creator/16, Bit_Multiplexer_2_to_1(02)/2, Logical Operator19/1
  Bus Selector/13 -> Logical Operator35/1, Bit_Multiplexer_2_to_1(09)/2  "<signal13>"
  Logical Operator35/1 -> Bit_Multiplexer_2_to_1(10)/2
  Bit_Multiplexer_2_to_1(09)/1 -> Bit_3/1
  Bit_Multiplexer_2_to_1(10)/1 -> Bit_3/3
  Logical Operator39/1 -> Bit_Multiplexer_2_to_1(07)/2
  Bus Selector/14 -> Logical Operator39/1, Bit_Multiplexer_2_to_1(06)/2  "<signal14>"
  Bit_Multiplexer_2_to_1(07)/1 -> Bit_2/3
  Bit_Multiplexer_2_to_1(06)/1 -> Bit_2/1
  Bus Selector/15 -> Logical Operator38/1, Bit_Multiplexer_2_to_1(03)/2  "<signal15>"
  Logical Operator38/1 -> Bit_Multiplexer_2_to_1(04)/2
  Bit_Multiplexer_2_to_1(04)/1 -> Bit_1/3
  Bit_Multiplexer_2_to_1(03)/1 -> Bit_1/1
  Logical Operator36/1 -> Bit_Multiplexer_2_to_1(01)/2
  Bit_Multiplexer_2_to_1(00)/1 -> Bit_0/1
  Bit_Multiplexer_2_to_1(01)/1 -> Bit_0/3
  Bus Selector/16 -> Logical Operator36/1, Bit_Multiplexer_2_to_1(00)/2  "<signal16>"
  Addr(2B)/1 -> Bus Selector/1
  Bit_3/1 -> Bus Creator/13, Bit_Multiplexer_2_to_1(11)/2, Logical Operator22/1
  Bit_2/1 -> Bus Creator/14, Bit_Multiplexer_2_to_1(08)/2, Logical Operator21/1
  Bit_3/2 -> Terminator8/1
  Logical Operator33/1 -> Logical Operator34/1, Bit_Multiplexer_2_to_1(07)/3, Bit_Multiplexer_2_to_1(06)/3
  Bit_1/1 -> Bus Creator/15, Bit_Multiplexer_2_to_1(05)/2, Logical Operator20/1
  Increment Enabled2/1 -> Bit_Multiplexer_2_to_1(04)/3, Bit_Multiplexer_2_to_1(03)/3, Logical Operator33/1
  Bit_2/2 -> Terminator7/1
  Bit_1/2 -> Terminator6/1
  Bit_0/2 -> Terminator16/1
  or/1 -> Bit_Multiplexer_2_to_1(01)/3, Increment Enabled2/1, Bit_Multiplexer_2_to_1(00)/3
  Logical Operator19/1 -> Bit_Multiplexer_2_to_1(02)/3
  Logical Operator20/1 -> Bit_Multiplexer_2_to_1(05)/3
  Logical Operator21/1 -> Bit_Multiplexer_2_to_1(08)/3
  Logical Operator22/1 -> Bit_Multiplexer_2_to_1(11)/3
  Logical Operator23/1 -> Bit_Multiplexer_2_to_1(14)/3
  Logical Operator24/1 -> Bit_Multiplexer_2_to_1(17)/3
  Logical Operator26/1 -> Bit_Multiplexer_2_to_1(20)/3
  Logical Operator29/1 -> Logical Operator27/1
  Bit_Multiplexer_2_to_1(02)/1 -> Increment Enabled2/2
  Bit_Multiplexer_2_to_1(05)/1 -> Logical Operator33/2
  Bit_Multiplexer_2_to_1(08)/1 -> Logical Operator34/2
  Bit_Multiplexer_2_to_1(11)/1 -> Logical Operator18/2
  Bit_Multiplexer_2_to_1(14)/1 -> Increment Enabled3/2
  Bit_Multiplexer_2_to_1(17)/1 -> Logical Operator14/2
  Bit_Multiplexer_2_to_1(20)/1 -> Logical Operator25/2
  Logical Operator28/1 -> or/1
  Logical Operator30/1 -> or/2
  Logical Operator31/1 -> Logical Operator28/1
  Decr(1b)/1 -> Logical Operator32/1, Logical Operator28/2, Logical Operator29/1
  Incr(1b)/1 -> Logical Operator27/2, Logical Operator30/1, Logical Operator31/1
  Logical Operator32/1 -> Logical Operator30/2
  Bus Creator/1 -> Bit to Integer Converter15/1, AddrOut(2B)/1
  Logical Operator5/1 -> Increment Enabled1/1, Bit_Multiplexer_2_to_1(25)/3, Bit_Multiplexer_2_to_1(24)/3
  Bus Selector/8 -> Bit_Multiplexer_2_to_1(24)/2, Logical Operator4/1  "<signal8>"
  Logical Operator4/1 -> Bit_Multiplexer_2_to_1(25)/2
  Bit_8/1 -> Bus Creator/8, Bit_Multiplexer_2_to_1(26)/2, Logical Operator7/1
  Bus Selector/5 -> Bit_Multiplexer_2_to_1(33)/2, Logical Operator11/1  "<signal5>"
  Logical Operator11/1 -> Bit_Multiplexer_2_to_1(34)/2
  Bit_Multiplexer_2_to_1(33)/1 -> Bit_11/1
  Bit_Multiplexer_2_to_1(34)/1 -> Bit_11/3
  Logical Operator3/1 -> Bit_Multiplexer_2_to_1(31)/2
  Bus Selector/6 -> Bit_Multiplexer_2_to_1(30)/2, Logical Operator3/1  "<signal6>"
  Bit_Multiplexer_2_to_1(31)/1 -> Bit_10/3
  Bit_Multiplexer_2_to_1(30)/1 -> Bit_10/1
  Bus Selector/7 -> Bit_Multiplexer_2_to_1(27)/2, Logical Operator2/1  "<signal7>"
  Logical Operator2/1 -> Bit_Multiplexer_2_to_1(28)/2
  Bit_Multiplexer_2_to_1(28)/1 -> Bit_9/3
  Bit_Multiplexer_2_to_1(27)/1 -> Bit_9/1
  SetDirect(1b)/1 -> Bit_Multiplexer_2_to_1(01)/1, Bit_Multiplexer_2_to_1(00)/1, Bit_Multiplexer_2_to_1(04)/1, Bit_Multiplexer_2_to_1(03)/1, Bit_Multiplexer_2_to_1(07)/1, Bit_Multiplexer_2_to_1(06)/1, Bit_Multiplexer_2_to_1(10)/1, Bit_Multiplexer_2_to_1(09)/1, Bit_Multiplexer_2_to_1(13)/1, Bit_Multiplexer_2_to_1(12)/1, Bit_Multiplexer_2_to_1(16)/1, Bit_Multiplexer_2_to_1(15)/1, Bit_Multiplexer_2_to_1(19)/1, Bit_Multiplexer_2_to_1(18)/1, Bit_Multiplexer_2_to_1(22)/1, Bit_Multiplexer_2_to_1(21)/1, Bit_Multiplexer_2_to_1(25)/1, Bit_Multiplexer_2_to_1(24)/1, Bit_Multiplexer_2_to_1(28)/1, Bit_Multiplexer_2_to_1(27)/1, Bit_Multiplexer_2_to_1(31)/1, Bit_Multiplexer_2_to_1(30)/1, Bit_Multiplexer_2_to_1(34)/1, Bit_Multiplexer_2_to_1(33)/1
  Bit_Multiplexer_2_to_1(24)/1 -> Bit_8/1
  Bit_Multiplexer_2_to_1(25)/1 -> Bit_8/3
  Bit_11/1 -> Bus Creator/5
  Bit_10/1 -> Bus Creator/6, Bit_Multiplexer_2_to_1(32)/2, Logical Operator10/1
  Logical Operator9/1 -> Bit_Multiplexer_2_to_1(34)/3, Bit_Multiplexer_2_to_1(33)/3
  Bit_11/2 -> Terminator2/1
  Logical Operator1/1 -> Logical Operator9/1, Bit_Multiplexer_2_to_1(31)/3, Bit_Multiplexer_2_to_1(30)/3
  Bit_9/1 -> Bus Creator/7, Bit_Multiplexer_2_to_1(29)/2, Logical Operator8/1
  Increment Enabled1/1 -> Logical Operator1/1, Bit_Multiplexer_2_to_1(28)/3, Bit_Multiplexer_2_to_1(27)/3
  Bit_10/2 -> Terminator1/1
  Clock/1 -> Bit_0/2, Bit_1/2, Bit_2/2, Bit_3/2, Bit_4/2, Bit_5/2, Bit_6/2, Bit_7/2, Bit_8/2, Bit_9/2, Bit_10/2, Bit_11/2
  Bit_9/2 -> Terminator4/1
  Bit_8/2 -> Terminator3/1
  Logical Operator25/1 -> Logical Operator5/1, Bit_Multiplexer_2_to_1(22)/3, Bit_Multiplexer_2_to_1(21)/3
  Logical Operator7/1 -> Bit_Multiplexer_2_to_1(26)/3
  Logical Operator8/1 -> Bit_Multiplexer_2_to_1(29)/3
  Logical Operator10/1 -> Bit_Multiplexer_2_to_1(32)/3
  Bit_Multiplexer_2_to_1(23)/1 -> Logical Operator5/2
  Bit_Multiplexer_2_to_1(26)/1 -> Increment Enabled1/2
  Bit_Multiplexer_2_to_1(29)/1 -> Logical Operator1/2
  Bit_Multiplexer_2_to_1(32)/1 -> Logical Operator9/2
  Logical Operator27/1 -> Bit_Multiplexer_2_to_1(02)/1, Bit_Multiplexer_2_to_1(05)/1, Bit_Multiplexer_2_to_1(08)/1, Bit_Multiplexer_2_to_1(11)/1, Bit_Multiplexer_2_to_1(14)/1, Bit_Multiplexer_2_to_1(17)/1, Bit_Multiplexer_2_to_1(20)/1, Bit_Multiplexer_2_to_1(23)/1, Bit_Multiplexer_2_to_1(26)/1, Bit_Multiplexer_2_to_1(32)/1, Bit_Multiplexer_2_to_1(29)/1
  Bus Selector/4 -> Terminator9/1  "<signal4>"
  Bus Selector/3 -> Terminator10/1  "<signal3>"
  Bus Selector/2 -> Terminator11/1  "<signal2>"
  Bus Selector/1 -> Terminator12/1  "<signal1>"
  Constant10/1 -> Bus Creator/1, Bus Creator/2, Bus Creator/3, Bus Creator/4
  Logical Operator6/1 -> Bit_Multiplexer_2_to_1(23)/3
  Bit to Integer Converter15/1 -> [STACK_POINTER]

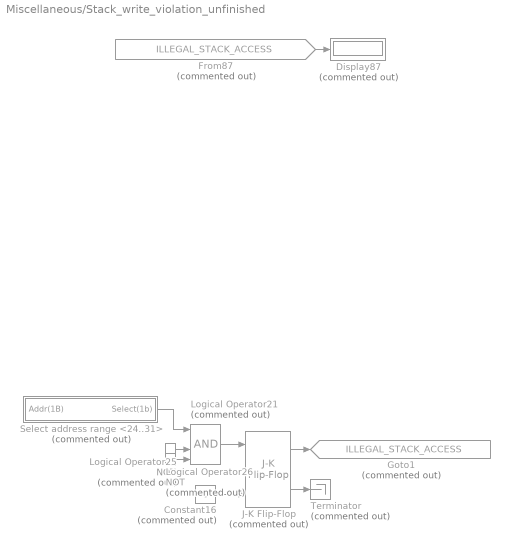
== system Miscellaneous/Stack_write_violation_unfinished ==
  Constant16 : Constant  Commented=on  Value=0  OutDataTypeStr=boolean
  Display87 : Display  Commented=on
      settings: Decimation=4
  From87 : From  Commented=on  GotoTag=ILLEGAL_STACK_ACCESS  TagVisibility=global
  Goto1 : Goto  Commented=on  GotoTag=ILLEGAL_STACK_ACCESS  TagVisibility=global
  J-K Flip-Flop : simulink_extras/Flip Flops/J-K Flip-Flop  Commented=on  initial_condition=0
  Logical Operator21 : Logic  Commented=on  Inputs=4  IconShape=distinctive  AllPortsSameDT=off  OutDataTypeStr=boolean
  Logical Operator25 : Logic  Commented=on  Operator=NOT  Inputs=1  IconShape=distinctive  AllPortsSameDT=off  OutDataTypeStr=boolean
  Logical Operator26 : Logic  Commented=on  Operator=NOT  Inputs=1  IconShape=distinctive  AllPortsSameDT=off  OutDataTypeStr=boolean
  Select address range <24..31> : Subsystem  Commented=on
  Terminator : Terminator  Commented=on
  wires:
  ? -> J-K Flip-Flop/2
  ? -> Logical Operator21/2
  ? -> Select address range <24..31>/1(Addr(1B))
  Logical Operator25/1 -> Logical Operator21/3
  ? -> Logical Operator25/1
  Select address range <24..31>/1(Select(1b)) -> Logical Operator21/1
  J-K Flip-Flop/2 -> Terminator/1
  Logical Operator21/1 -> J-K Flip-Flop/1
  J-K Flip-Flop/1 -> Goto1/1
  Constant16/1 -> J-K Flip-Flop/3
  Logical Operator26/1 -> Logical Operator21/4
  ? -> Logical Operator26/1
  From87/1 -> Display87/1

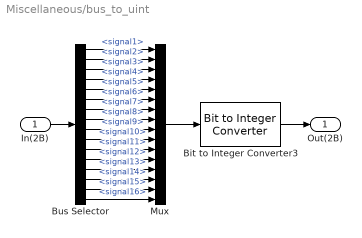
== system Miscellaneous/bus_to_uint ==
  In(2B) : Inport
  Bit to Integer Converter3 : commutil2/Bit to Integer Converter  nbits=16  bitOrder=MSB first  signedOutputValues=Unsigned  outDtype=uint16  outDtypeSigned=Inherit via internal rule
  Bus Selector : BusSelector  OutputSignals=signal1,signal2,signal3,signal4,signal5,signal6,signal7,signal8,signal9,signal10,signal11,signal12,signal13,signal14,signal15,signal16
  Mux : Mux  Inputs=16
  Out(2B) : Outport
  wires:
  In(2B)/1 -> Bus Selector/1
  Bit to Integer Converter3/1 -> Out(2B)/1
  Bus Selector/1 -> Mux/1  "<signal1>"
  Bus Selector/2 -> Mux/2  "<signal2>"
  Bus Selector/3 -> Mux/3  "<signal3>"
  Bus Selector/4 -> Mux/4  "<signal4>"
  Bus Selector/5 -> Mux/5  "<signal5>"
  Bus Selector/6 -> Mux/6  "<signal6>"
  Bus Selector/7 -> Mux/7  "<signal7>"
  Bus Selector/8 -> Mux/8  "<signal8>"
  Bus Selector/10 -> Mux/10  "<signal10>"
  Bus Selector/9 -> Mux/9  "<signal9>"
  Bus Selector/11 -> Mux/11  "<signal11>"
  Bus Selector/12 -> Mux/12  "<signal12>"
  Bus Selector/13 -> Mux/13  "<signal13>"
  Bus Selector/14 -> Mux/14  "<signal14>"
  Bus Selector/15 -> Mux/15  "<signal15>"
  Bus Selector/16 -> Mux/16  "<signal16>"
  Mux/1 -> Bit to Integer Converter3/1

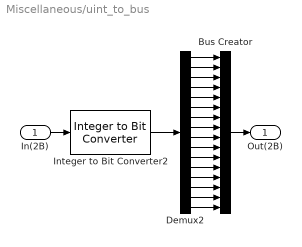
== system Miscellaneous/uint_to_bus ==
  In(2B) : Inport
  Bus Creator : BusCreator  Inputs=16
  Demux2 : Demux  Outputs=16
  Integer to Bit Converter2 : commutil2/Integer to Bit Converter  nbits=16  signedInputValues=Unsigned  bitOrder=MSB first  outDtype=boolean
  Out(2B) : Outport
  wires:
  In(2B)/1 -> Integer to Bit Converter2/1
  Bus Creator/1 -> Out(2B)/1
  Demux2/13 -> Bus Creator/13
  Demux2/1 -> Bus Creator/1
  Demux2/5 -> Bus Creator/5
  Demux2/16 -> Bus Creator/16
  Demux2/3 -> Bus Creator/3
  Demux2/11 -> Bus Creator/11
  Demux2/12 -> Bus Creator/12
  Demux2/15 -> Bus Creator/15
  Demux2/14 -> Bus Creator/14
  Demux2/2 -> Bus Creator/2
  Demux2/6 -> Bus Creator/6
  Demux2/9 -> Bus Creator/9
  Demux2/10 -> Bus Creator/10
  Demux2/4 -> Bus Creator/4
  Demux2/7 -> Bus Creator/7
  Demux2/8 -> Bus Creator/8
  Integer to Bit Converter2/1 -> Demux2/1

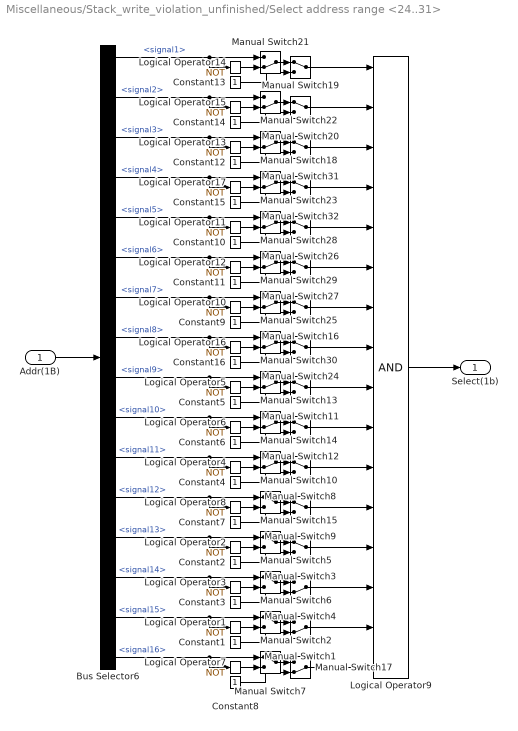
== system Miscellaneous/Stack_write_violation_unfinished/Select address range <24..31> ==
  Addr(1B) : Inport
  Bus Selector6 : BusSelector  OutputSignals=signal1,signal2,signal3,signal4,signal5,signal6,signal7,signal8,signal9,signal10,signal11,signal12,signal13,signal14,signal15,signal16
  Constant{1..16} (16 alike) : Constant  OutDataTypeStr=boolean
  Logical Operator{1..8,10..17} (16 alike) : Logic  Operator=NOT  Inputs=1  IconShape=distinctive  AllPortsSameDT=off  OutDataTypeStr=boolean
  Logical Operator9 : Logic  Inputs=16  IconShape=distinctive  AllPortsSameDT=off  OutDataTypeStr=boolean
  Manual Switch{1,4,10,13..14,17..18,21..23,25,28..30} (14 alike) : ManualSwitch  CurrentSetting=0
  Manual Switch{2..3,5..9,11..12,15..16,19..20,24,26..27,31..32} (18 alike) : ManualSwitch
  Select(1b) : Outport
  wires:
  Logical Operator7/1 -> Manual Switch7/2
  Bus Selector6/16 -> Logical Operator7/1, Manual Switch7/1  "<signal16>"
  Manual Switch17/1 -> Logical Operator9/16
  Manual Switch7/1 -> Manual Switch17/1
  Constant8/1 -> Manual Switch17/2
  Logical Operator9/1 -> Select(1b)/1
  Logical Operator1/1 -> Manual Switch2/2
  Bus Selector6/15 -> Logical Operator1/1, Manual Switch2/1  "<signal15>"
  Manual Switch1/1 -> Logical Operator9/15
  Manual Switch2/1 -> Manual Switch1/1
  Constant1/1 -> Manual Switch1/2
  Addr(1B)/1 -> Bus Selector6/1
  Logical Operator3/1 -> Manual Switch6/2
  Bus Selector6/14 -> Logical Operator3/1, Manual Switch6/1  "<signal14>"
  Manual Switch4/1 -> Logical Operator9/14
  Manual Switch6/1 -> Manual Switch4/1
  Constant3/1 -> Manual Switch4/2
  Logical Operator2/1 -> Manual Switch5/2
  Bus Selector6/13 -> Logical Operator2/1, Manual Switch5/1  "<signal13>"
  Manual Switch3/1 -> Logical Operator9/13
  Manual Switch5/1 -> Manual Switch3/1
  Constant2/1 -> Manual Switch3/2
  Logical Operator8/1 -> Manual Switch15/2
  Bus Selector6/12 -> Logical Operator8/1, Manual Switch15/1  "<signal12>"
  Manual Switch9/1 -> Logical Operator9/12
  Manual Switch15/1 -> Manual Switch9/1
  Constant7/1 -> Manual Switch9/2
  Logical Operator4/1 -> Manual Switch10/2
  Bus Selector6/11 -> Logical Operator4/1, Manual Switch10/1  "<signal11>"
  Manual Switch8/1 -> Logical Operator9/11
  Manual Switch10/1 -> Manual Switch8/1
  Constant4/1 -> Manual Switch8/2
  Logical Operator6/1 -> Manual Switch14/2
  Bus Selector6/10 -> Logical Operator6/1, Manual Switch14/1  "<signal10>"
  Manual Switch12/1 -> Logical Operator9/10
  Manual Switch14/1 -> Manual Switch12/1
  Constant6/1 -> Manual Switch12/2
  Logical Operator5/1 -> Manual Switch13/2
  Bus Selector6/9 -> Logical Operator5/1, Manual Switch13/1  "<signal9>"
  Manual Switch11/1 -> Logical Operator9/9
  Manual Switch13/1 -> Manual Switch11/1
  Constant5/1 -> Manual Switch11/2
  Logical Operator16/1 -> Manual Switch30/2
  Bus Selector6/8 -> Logical Operator16/1, Manual Switch30/1  "<signal8>"
  Manual Switch24/1 -> Logical Operator9/8
  Manual Switch30/1 -> Manual Switch24/1
  Constant16/1 -> Manual Switch24/2
  Logical Operator10/1 -> Manual Switch25/2
  Bus Selector6/7 -> Logical Operator10/1, Manual Switch25/1  "<signal7>"
  Manual Switch16/1 -> Logical Operator9/7
  Manual Switch25/1 -> Manual Switch16/1
  Constant9/1 -> Manual Switch16/2
  Logical Operator12/1 -> Manual Switch29/2
  Bus Selector6/6 -> Logical Operator12/1, Manual Switch29/1  "<signal6>"
  Manual Switch27/1 -> Logical Operator9/6
  Manual Switch29/1 -> Manual Switch27/1
  Constant11/1 -> Manual Switch27/2
  Logical Operator11/1 -> Manual Switch28/2
  Bus Selector6/5 -> Logical Operator11/1, Manual Switch28/1  "<signal5>"
  Manual Switch26/1 -> Logical Operator9/5
  Manual Switch28/1 -> Manual Switch26/1
  Constant10/1 -> Manual Switch26/2
  Logical Operator17/1 -> Manual Switch23/2
  Bus Selector6/4 -> Logical Operator17/1, Manual Switch23/1  "<signal4>"
  Manual Switch32/1 -> Logical Operator9/4
  Manual Switch23/1 -> Manual Switch32/1
  Constant15/1 -> Manual Switch32/2
  Logical Operator13/1 -> Manual Switch18/2
  Bus Selector6/3 -> Logical Operator13/1, Manual Switch18/1  "<signal3>"
  Manual Switch31/1 -> Logical Operator9/3
  Manual Switch18/1 -> Manual Switch31/1
  Constant12/1 -> Manual Switch31/2
  Logical Operator15/1 -> Manual Switch22/2
  Bus Selector6/2 -> Logical Operator15/1, Manual Switch22/1  "<signal2>"
  Manual Switch20/1 -> Logical Operator9/2
  Manual Switch22/1 -> Manual Switch20/1
  Constant14/1 -> Manual Switch20/2
  Logical Operator14/1 -> Manual Switch21/2
  Bus Selector6/1 -> Logical Operator14/1, Manual Switch21/1  "<signal1>"
  Manual Switch19/1 -> Logical Operator9/1
  Manual Switch21/1 -> Manual Switch19/1
  Constant13/1 -> Manual Switch19/2
